simulink model "hoppingControl"  (R2018b)
settings: Solver=FixedStepAuto  StartTime=0.0  StopTime=inf  RelTol=1e-3  EnableMultiTasking=on
libraries: dspstat3 x19, cm_custom x9, raspberrypilib x8, simulink_extras x3, peGeneralControl x3, can_bus_multi x2, simulink x1, embdlinuxlib x1
(part 1 of 3)
settings Model: SimulationMode=external  Creator=Ivan Fan  LastModifiedBy=User
settings SolverCC: PositivePriorityOrder=on
settings OptimizationCC: EnhancedBackFolding=on  PassReuseOutputArgsThreshold=0  MaxStackSize=64  OptimizeBlockOrder=speed  DifferentSizesBufferReuse=on
settings DebuggingCC: ParameterTunabilityLossMsg=error  UnderSpecifiedDimensionMsg=error
settings HardwareCC: ProdBitPerPointer=32  ProdBitPerSizeT=32  ProdBitPerPtrDiffT=32  ProdLargestAtomicInteger=Long  ProdLargestAtomicFloat=Double  ProdWordSize=32  ProdHWDeviceType=ARM Compatible->ARM Cortex  UseEmbeddedCoderFeatures=off
settings SFSimCC: MATLABDynamicMemAlloc=off
settings RTWCC: SystemTargetFile=ert.tlc  HardwareBoard=Raspberry Pi  TLCOptions="-aInlineSetEventsForThisBaseRateFcn=TLC_FALSE -aSuppressMultiTaskScheduler=TLC_FALSE  -aRateBasedStepFcn=0"  TemplateMakefile=ert_default_tmf  GenerateReport=on  Toolchain=GNU GCC Raspberry Pi  BuildConfiguration=Faster Runs  LaunchReport=on  TargetLang=C++
settings CodeAppCC: ForceParamTrailComments=on  OperatorAnnotations=on
settings ERTTargetCC: TargetLangStandard=C++03 (ISO)  ERTCustomFileBanners=off  SupportContinuousTime=on  SupportNonInlinedSFcns=on  RemoveResetFunc=off  SupportVariableSizeSignals=on  ModelStepFunctionPrototypeControlCompliant=off  ExtMode=on  ExtModeMexArgs='192.168.137.181' 0 17725  ERTSrcFileBannerTemplate=codertarget_code_template.cgt  ERTHdrFileBannerTemplate=codertarget_code_template.cgt  ERTDataSrcFileTemplate=codertarget_code_template.cgt  ERTDataHdrFileTemplate=codertarget_code_template.cgt

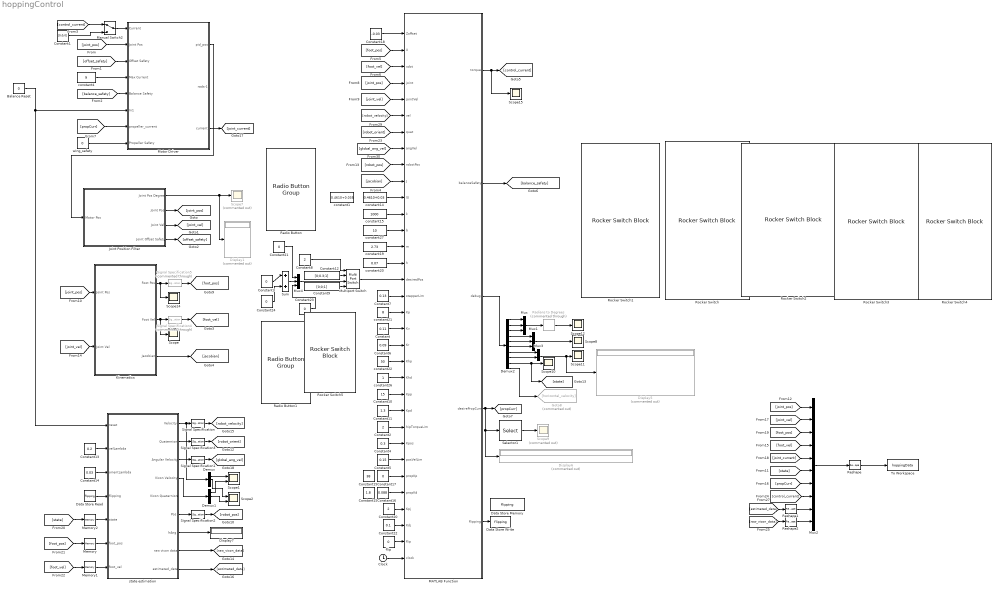
== system hoppingControl ==
  Balance Reset : Constant  Value=0
  Clock : Clock
  Constant : Constant  Value=0.11
  Constant1 : Constant  Value=[0;0;0]
  Constant10 : Constant  Value=15
  Constant11 : Constant  Value=1.3
  Constant12 : Constant  Value=[0;0.3;1]
  Constant13 : Constant  Value=0.2
  Constant14 : Constant  Value=0.03  VectorParams1D=off
  Constant15 : Constant  Value=1.8
  Constant16 : Constant  Value=0.088
  Constant{3,17,21,23..24} (5 alike) : Constant  Value=0
  Constant18 : Constant  Value=-0.03
  Constant19 : Constant  Value=38
  Constant2 : Constant  Value=2
  Constant20 : Constant  Value=2
  Constant22 : Constant  Value=0.1
  Constant4 : Constant  Value=0.3
  Constant5 : Constant  Value=0.15
  Constant6 : Constant  Value=0.09
  Constant7 : Constant  Value=0.13
  Constant8 : Constant  Value=2
  Constant9 : Constant  Value=[0;0;1]
  Data Store Memory : DataStoreMemory  DataStoreName=flipping  ReadBeforeWriteMsg=warning  WriteAfterWriteMsg=warning  WriteAfterReadMsg=warning  ShowAdditionalParam=off
  Data Store Read : DataStoreRead  DataStoreName=flipping
  Data Store Write : DataStoreWrite  DataStoreName=flipping
  Demux : Demux  Outputs=3
  Demux1 : Demux  Outputs=3
  Demux2 : Demux  Outputs=10
  Display1 : Display  Commented=on
      settings: Decimation=100
  Display5 : Display  Commented=on
  Display6 : Display  Commented=on
  Display7 : Display
  Goto8 : Goto  Commented=on  GotoTag=horizontal_velocity
  Joint Position Filter : Subsystem
  Kinematics : Subsystem
  MATLAB Function : MATLAB Function  TreatAsAtomicUnit=on
  Manual Switch2 : ManualSwitch
  Memory : Memory  InitialCondition=[0;0;0]
  Memory1 : Memory  InitialCondition=[0;0;0]
  Memory2 : Memory
  Motor Driver : Subsystem
  Multiport Switch : MultiPortSwitch
  Mux : Mux  Inputs=3
  Mux1 : Mux  Inputs=3
  Mux2 : Mux  Inputs=10
  Mux3 : Mux  Inputs=2
  Mux4 : Mux  Inputs=3
  Radians to Degrees : simulink_extras/Transformations/Radians to Degrees  Commented=through
  Radio Button : RadioButtonGroup  WebBlockId=1587  SelectedLabel=0  ButtonGroupName=x fine tune
      settings: Values={{'0.3', '0.2', '0.1', '0', '-0.1', '-0.2', '-0.3'}, [0.3 0.2 0.1 0 -0.1 -0.2 -0.3]}
  Radio Button1 : RadioButtonGroup  WebBlockId=1588  SelectedLabel=0  ButtonGroupName=y fine tune
      settings: Values={{'0.3', '0.2', '0.1', '0', '-0.1', '-0.2', '-0.3'}, [0.3 0.2 0.1 0 -0.1 -0.2 -0.3]}
  Reshape : Reshape
  Reshape1 : Reshape  OutputDimensionality=Column vector (2-D)
  Reshape2 : Reshape  OutputDimensionality=Column vector (2-D)
  Rocker Switch : RockerSwitchBlock  WebBlockId=606
      settings: Values={{'Off', 'On'}, [0 1]}
  Rocker Switch1 : RockerSwitchBlock  WebBlockId=618
      settings: Values={{'Off', 'On'}, [0 1]}
  Rocker Switch2 : RockerSwitchBlock  WebBlockId=667
      settings: Values={{'Off', 'On'}, [0 1]}
  Rocker Switch3 : RockerSwitchBlock  WebBlockId=1032
      settings: Values={{'Off', 'On'}, [0 1]}
  Rocker Switch4 : RockerSwitchBlock  WebBlockId=1024
      settings: Values={{'Off', 'On'}, [0 1]}
  Rocker Switch5 : RockerSwitchBlock  WebBlockId=1531
      settings: Values={{'Off', 'On'}, [-8 0]}
  Scope{,8,10..12,14..15} (7 alike) : Scope
  Scope1 : Scope  NumInputPorts=2
  Scope2 : Scope  NumInputPorts=2
  Scope7 : Scope  Commented=on
  Scope9 : Scope  Commented=on
  Selector1 : Selector  InputPortWidth=4  IndexOptions=Index vector (dialog)  Indices=[2 3 4]  OutputSizes=1
  Signal Specification : SignalSpecification  Dimensions=3
  Signal Specification1 : SignalSpecification  Dimensions=3
  Signal Specification2 : SignalSpecification  Dimensions=3
  Signal Specification3 : SignalSpecification  Dimensions=4
  Signal Specification4 : SignalSpecification  Commented=through  Dimensions=[3 1]
  Signal Specification5 : SignalSpecification  Commented=through  Dimensions=[3 1]
  Sum : Sum  Inputs=|++
  To Workspace : ToWorkspace  VariableName=hoppingData  SampleTime=-1
      settings: Save2DSignal=2-D array (concatenate along first dimension)
  constant1 : Constant  Value=0.4610+0.035
  constant14 : Constant  Value=0.4610+0.03
  constant15 : Constant  Value=1000
  constant19 : Constant  Value=2.73
  constant20 : Constant  Value=0.07
  constant21 : Constant  Value=8
  constant22 : Constant  Value=50
  constant26 : Constant
  constant27 : Constant  Value=10
  constant4 : Constant  Value=9
  flip : Constant  Value=0
  state estimation : Subsystem
  wing_safety : Constant  Value=0
  wires:
  Constant1/1 -> Manual Switch2/2
  Manual Switch2/1 -> Motor Driver/1(Current)
  Joint Position Filter/1(Joint Pos Degree) -> Scope7/1, Display1/1
  Joint Position Filter/2(Joint Pos) -> [joint_pos]
  Joint Position Filter/3(Joint Vel) -> [joint_vel]
  [joint_pos] -> Motor Driver/2(Joint Pos)
  [offset_safety] -> Motor Driver/3(Offset Safety)
  constant4/1 -> Motor Driver/4(Max Current)
  [balance_safety] -> Motor Driver/5(Balance Safety)
  [control_current] -> Manual Switch2/1
  Kinematics/2(Foot Vel) -> Signal Specification4/1, Scope/1
  [joint_pos] -> Kinematics/1(Joint Pos)
  [joint_vel] -> Kinematics/2(Joint Vel)
  [jacobian] -> MATLAB Function/10(J)
  [foot_pos] -> MATLAB Function/2(X)
  Constant18/1 -> MATLAB Function/1(Zoffset)
  [foot_vel] -> MATLAB Function/3(xdot)
  constant14/1 -> MATLAB Function/11(l0)
  constant27/1 -> MATLAB Function/13(b)
  constant15/1 -> MATLAB Function/12(k)
  constant19/1 -> MATLAB Function/14(m)
  constant20/1 -> MATLAB Function/15(h)
  Constant7/1 -> MATLAB Function/17(stepperLim)
  constant21/1 -> MATLAB Function/18(Kp)
  constant22/1 -> MATLAB Function/21(Khp)
  constant26/1 -> MATLAB Function/22(Khd)
  Constant6/1 -> MATLAB Function/20(Kr)
  Constant/1 -> MATLAB Function/19(Kv)
  MATLAB Function/1(torque) -> Scope15/1, [control_current]
  MATLAB Function/2(balanceSafety) -> [balance_safety]
  Kinematics/3(Jacobian) -> [jacobian]
  Constant10/1 -> MATLAB Function/23(Kpp)
  Constant11/1 -> MATLAB Function/24(Kpd)
  Constant2/1 -> MATLAB Function/25(hipTorqueLim)
  Balance Reset/1 -> Motor Driver/6(In1), state estimation/1(reset)
  MATLAB Function/3(debug) -> Demux2/1
  state estimation/4(Vicon Velocity) -> Demux1/1
  Demux/1 -> Scope1/1
  Demux1/1 -> Scope1/2
  Demux/2 -> Scope2/1
  Demux1/2 -> Scope2/2
  Constant4/1 -> MATLAB Function/26(Kpos)
  Constant5/1 -> MATLAB Function/27(posVelLim)
  Constant8/1 -> Multiport Switch/1
  Constant9/1 -> Multiport Switch/4
  Constant12/1 -> Multiport Switch/2
  Constant14/1 -> state estimation/3(orientLambda)
  Constant13/1 -> state estimation/2(velLambda)
  [propCurr] -> Motor Driver/7(propeller_current)
  Constant17/1 -> MATLAB Function/28(propKp)
  Demux2/5 -> Mux1/2
  Demux2/4 -> Mux1/1
  Demux2/3 -> Mux/3
  Demux2/2 -> Mux/2
  Demux2/1 -> Mux/1
  Mux/1 -> Radians to Degrees/1
  Constant16/1 -> MATLAB Function/29(propKd)
  Demux2/6 -> Mux1/3
  Multiport Switch/1 -> MATLAB Function/16(desiredPos)
  Demux2/9 -> [state], Scope10/1
  Demux2/7 -> Mux3/1
  Demux2/8 -> Mux3/2
  Demux2/10 -> Goto8/1
  MATLAB Function/4(desirePropCurr) -> Display6/1, Selector1/1, [propCurr]
  [joint_pos] -> MATLAB Function/4(joint)
  [joint_vel] -> MATLAB Function/5(jointVel)
  Clock/1 -> MATLAB Function/33(clock)
  Constant20/1 -> MATLAB Function/30(Kpj)
  Constant22/1 -> MATLAB Function/31(Kdj)
  Mux1/1 -> Scope8/1
  wing_safety/1 -> Motor Driver/8(Propeller Safety)
  flip/1 -> MATLAB Function/32(flip)
  MATLAB Function/5(flipping) -> Data Store Write/1
  Data Store Read/1 -> state estimation/4(flipping)
  Radians to Degrees/1 -> Scope12/1
  Selector1/1 -> Scope9/1
  Mux3/1 -> Display5/1, Scope11/1
  [robot_pos] -> MATLAB Function/9(robotPos)
  [joint_pos] -> Mux2/1
  [joint_vel] -> Mux2/2
  Mux2/1 -> Reshape/1
  [state] -> Mux2/6
  Joint Position Filter/4(Joint Offset Safety) -> [offset_safety]
  Motor Driver/1(pid_pos) -> Joint Position Filter/1(Motor Pos)
  [foot_pos] -> Mux2/3
  [state] -> Memory2/1
  [foot_pos] -> Memory/1
  [foot_vel] -> Memory1/1
  Kinematics/1(Foot Pos) -> Signal Specification5/1, Scope14/1
  Memory/1 -> state estimation/6(foot_pos)
  Memory1/1 -> state estimation/7(foot_vel)
  Memory2/1 -> state estimation/5(state)
  state estimation/6(Pos) -> Signal Specification2/1
  state estimation/3(Angular Velocity) -> Signal Specification1/1
  state estimation/1(Velocity) -> Demux/1, Signal Specification/1
  state estimation/2(Quaternion) -> Signal Specification3/1
  Signal Specification/1 -> [robot_velocity]
  Signal Specification1/1 -> [global_ang_vel]
  Signal Specification2/1 -> [robot_pos]
  Signal Specification3/1 -> [robot_orient]
  [robot_orient] -> MATLAB Function/7(quat)
  Signal Specification4/1 -> [foot_vel]
  Signal Specification5/1 -> [foot_pos]
  state estimation/7(hAng) -> Display7/1
  state estimation/8(raw vicon data) -> [raw_vicon_data]
  [control_current] -> Mux2/8
  Reshape/1 -> To Workspace/1
  [raw_vicon_data] -> Reshape2/1
  state estimation/9(estimated_data) -> [estimated_data]
  [estimated_data] -> Reshape1/1
  Motor Driver/3(current) -> [joint_current]
  Constant23/1 -> Mux4/3
  Constant21/1 -> Mux4/1
  Constant3/1 -> Sum/1
  Mux4/1 -> Multiport Switch/3
  [robot_velocity] -> MATLAB Function/6(vel)
  [global_ang_vel] -> MATLAB Function/8(angVel)
  [foot_vel] -> Mux2/4
  [propCurr] -> Mux2/7
  [joint_current] -> Mux2/5
  Reshape1/1 -> Mux2/9
  Reshape2/1 -> Mux2/10
  Constant24/1 -> Sum/2
  Sum/1 -> Mux4/2

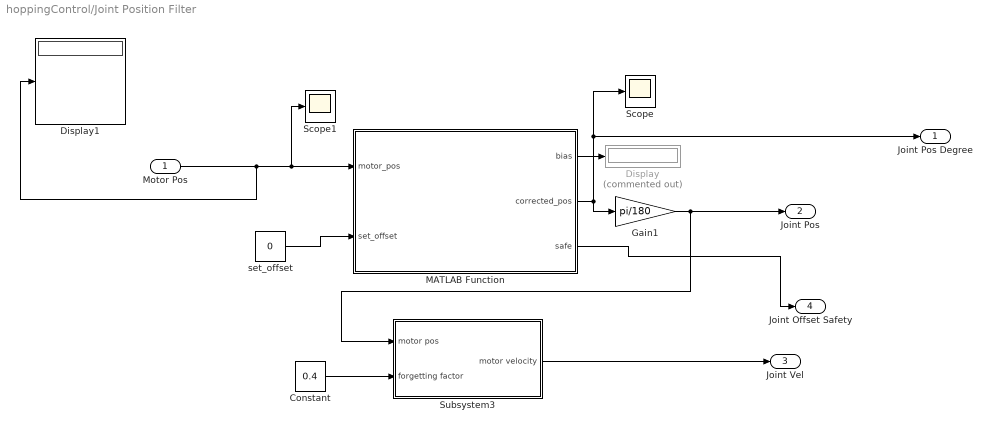
== system hoppingControl/Joint Position Filter ==
  Motor Pos : Inport
  Constant : Constant  Value=0.4
  Display : Display  Commented=on
      settings: Decimation=100
  Display1 : Display
  Gain1 : Gain  Gain=pi/180
  MATLAB Function : MATLAB Function  TreatAsAtomicUnit=on
  Scope : Scope
  Scope1 : Scope
  Subsystem3 : Subsystem
  set_offset : Constant  Value=0
  Joint Pos Degree : Outport
  Joint Pos : Outport  Port=2
  Joint Vel : Outport  Port=3
  Joint Offset Safety : Outport  Port=4
  wires:
  Subsystem3/1("motor velocity ") -> Joint Vel/1
  MATLAB Function/2(corrected_pos) -> Scope/1, Joint Pos Degree/1, Gain1/1
  MATLAB Function/1(bias) -> Display/1
  set_offset/1 -> MATLAB Function/2(set_offset)
  Constant/1 -> Subsystem3/2(forgetting factor)
  Motor Pos/1 -> Display1/1, Scope1/1, MATLAB Function/1(motor_pos)
  MATLAB Function/3(safe) -> Joint Offset Safety/1
  Gain1/1 -> Subsystem3/1(motor pos), Joint Pos/1

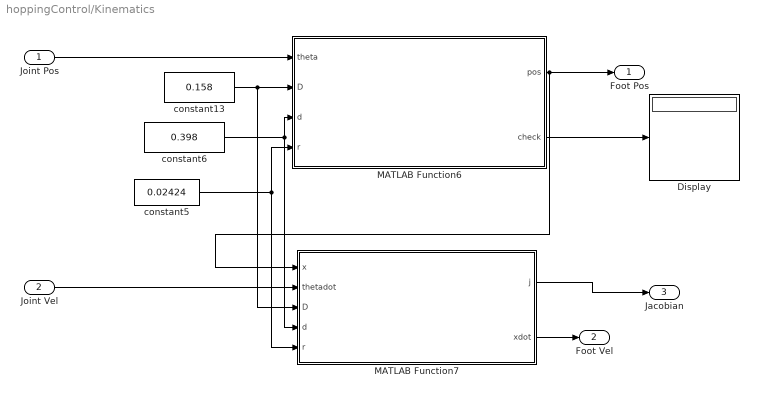
== system hoppingControl/Kinematics ==
  Joint Pos : Inport
  Joint Vel : Inport  Port=2
  Display : Display
      settings: Decimation=100
  MATLAB Function6 : MATLAB Function  TreatAsAtomicUnit=on
  MATLAB Function7 : MATLAB Function  TreatAsAtomicUnit=on
  constant13 : Constant  Value=0.158
  constant5 : Constant  Value=0.02424
  constant6 : Constant  Value=0.398
  Foot Pos : Outport
  Foot Vel : Outport  Port=2
  Jacobian : Outport  Port=3
  wires:
  constant6/1 -> MATLAB Function7/4(d), MATLAB Function6/3(d)
  constant5/1 -> MATLAB Function7/5(r), MATLAB Function6/4(r)
  constant13/1 -> MATLAB Function6/2(D), MATLAB Function7/3(D)
  Joint Pos/1 -> MATLAB Function6/1(theta)
  MATLAB Function7/1(j) -> Jacobian/1
  MATLAB Function6/2(check) -> Display/1
  Joint Vel/1 -> MATLAB Function7/2(thetadot)
  MATLAB Function6/1(pos) -> MATLAB Function7/1(x), Foot Pos/1
  MATLAB Function7/2(xdot) -> Foot Vel/1

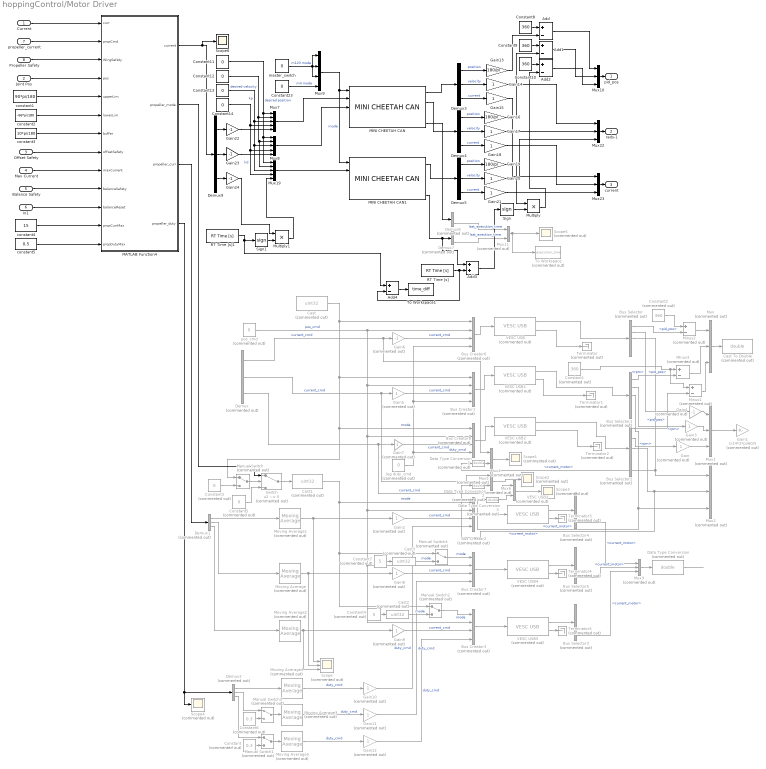
== system hoppingControl/Motor Driver ==
  Current : Inport
  Joint Pos : Inport  Port=2
  Offset Safety : Inport  Port=3
  Max Current : Inport  Port=4
  Balance Safety : Inport  Port=5
  In1 : Inport  Port=6
  propeller_current : Inport  Port=7
  Propeller Safety : Inport  Port=8
  Add{,1..2,4} (4 alike) : Sum  Inputs=+-
  Add3 : Sum
  Bus Creator{1..3,6..8} (6 alike) : BusCreator  Commented=on  Inputs=4
  Bus Selector : BusSelector  Commented=on  OutputSignals=pid_pos,rpm,current_motor,v_in,fault_code
  Bus Selector1 : BusSelector  Commented=on  OutputSignals=pid_pos,rpm,current_motor,v_in,fault_code
  Bus Selector2 : BusSelector  Commented=on  OutputSignals=pid_pos,rpm,current_motor,v_in,fault_code
  Bus Selector3 : BusSelector  Commented=on  OutputSignals=pid_pos,rpm,current_motor
  Bus Selector4 : BusSelector  Commented=on  OutputSignals=pid_pos,rpm,current_motor
  Bus Selector5 : BusSelector  Commented=on  OutputSignals=pid_pos,rpm,current_motor
  Cast{,1..3} (4 alike) : DataTypeConversion  Commented=on  OutDataTypeStr=uint32  RndMeth=Round
  Cast To Double : DataTypeConversion  Commented=on  OutDataTypeStr=double
  Constant : Constant  Commented=on  Value=0.3
  Constant1 : Constant  Commented=on  Value=360  OutDataTypeStr=Inherit: Inherit via back propagation
  Constant10 : Constant  Value=360
  Constant{11..14,23} (5 alike) : Constant  Value=0
  Constant2 : Constant  Commented=on  Value=360  OutDataTypeStr=Inherit: Inherit via back propagation
  Constant3 : Constant  Commented=on  Value=0
  Constant4 : Constant  Commented=on  Value=5
  Constant5 : Constant  Commented=on  Value=0
  Constant6 : Constant  Commented=on  Value=0.3
  Constant7 : Constant  Commented=on  Value=5
  Constant8 : Constant  Value=360
  Constant9 : Constant  Value=360
  Data Type Conversion{,1..3} (4 alike) : DataTypeConversion  Commented=on  OutDataTypeStr=double
  Demux{,1..2,7..8} (5 alike) : Demux  Commented=on  Outputs=3
  Demux{3..5,9} (4 alike) : Demux  Outputs=3
  Gain{,3,5,7} (4 alike) : Gain  Commented=on  OutDataTypeStr=Inherit: Same as input
  Gain1 : Gain  Commented=on  Gain=1/14*2*pi/60/5  OutDataTypeStr=Inherit: Same as input
  Gain{2,8..12} (6 alike) : Gain  Commented=on
  Gain13 : Gain  Gain=180/pi
  Gain{14..15,17..18,20..21} (6 alike) : Gain
  Gain16 : Gain  Gain=180/pi
  Gain19 : Gain  Gain=180/pi
  Gain22 : Gain  Gain=-1
  Gain23 : Gain  Gain=-1
  Gain24 : Gain  Gain=-1
  Gain4 : Gain  Commented=on  Gain=-1  OutDataTypeStr=Inherit: Same as input
  Gain6 : Gain  Commented=on  Gain=-1  OutDataTypeStr=Inherit: Same as input
  MATLAB Function4 : MATLAB Function  TreatAsAtomicUnit=on
  MINI CHEETAH CAN : can_bus_multi/MINI CHEETAH CAN  PAR_PORT_NUM=can0  PAR_SAFE=on  PAR_DEV_NUM=3  PAR_SMPLT=0.002
      link override S-Function Builder: Parameters=uint8(PAR_DEV_NUM),uint8(PAR_PORT_NUM),uint8(PAR_SAFE)  FunctionName=CAN_BUS_MULTISTATE_SF  SFunctionModules=CAN_BUS_MULTISTATE_SF_wrapper
      settings: SourceProductName=CAN Bus Multi
  MINI CHEETAH CAN1 : can_bus_multi/MINI CHEETAH CAN  PAR_PORT_NUM=can1  PAR_SAFE=on  PAR_DEV_NUM=1  PAR_SMPLT=0.002
      link override S-Function Builder: Parameters=uint8(PAR_DEV_NUM),uint8(PAR_PORT_NUM),uint8(PAR_SAFE)  FunctionName=CAN_BUS_MULTISTATE_SF  SFunctionModules=CAN_BUS_MULTISTATE_SF_wrapper
      settings: SourceProductName=CAN Bus Multi
  Manual Switch{,1..4} (5 alike) : ManualSwitch  Commented=on
  Minus1 : Sum  Commented=on  Inputs=+-
  Minus2 : Sum  Commented=on  Inputs=+-
  Minus3 : Sum  Commented=on  Inputs=+-
  Moving Average{,1..5} (6 alike) : dspstat3/Moving Average  Commented=on  Method=Sliding window  ForgettingFactorPort=off  SpecifyWindowLength=on  WindowLength=4  ForgettingFactor=0.9  SimulateUsing=Code generation
  Multiply : Product
  Multiply1 : Product
  Mux{,1..3} (4 alike) : Mux  Commented=on  Inputs=3
  Mux10 : Mux  Inputs=3
  Mux{4..6,11} (4 alike) : Mux  Commented=on  Inputs=2
  Mux19 : Mux  Inputs=5
  Mux22 : Mux  Inputs=3
  Mux23 : Mux  Inputs=3
  Mux7 : Mux  Inputs=5
  Mux8 : Mux  Inputs=5
  Mux9 : Mux
  RT Time [s] : cm_custom/RT Time [s]
      settings: SourceProductName=cm custom
  RT Time [s]1 : cm_custom/RT Time [s]
      settings: SourceProductName=cm custom
  Scope : Scope  Commented=on  NumInputPorts=3
  Scope{1..5} (5 alike) : Scope  Commented=on
  Scope6 : Scope
  Sign : Signum
  Sign1 : Signum
  Switch : Switch  Commented=on  Criteria=u2 ~= 0
  Terminator{,1..5} (6 alike) : Terminator  Commented=on
  To Workspace : ToWorkspace  Commented=on  VariableName=execution_time  SampleTime=-1
  To Workspace1 : ToWorkspace  VariableName=time_diff  SampleTime=-1
      settings: Save2DSignal=2-D array (concatenate along first dimension)
  VESC USB : cm_custom/VESC USB  Commented=on  PAR_VESC_DEV='/dev/leg_a'  POS_KP=0.05  POS_KI=0  POS_KD=0.0008  POS_KD_FIL=0.8  POS_DIV=5  CURR_MAX=25  CURR_MIN=-25  CURR_IN_MAX=20  CURR_IN_MIN=-20  CURR_ABS_MAX=40  PAR_SMPLT=0.0015
      link override S-Function Builder5: Parameters=uint8(PAR_VESC_DEV)
      settings: SourceProductName=cm custom
  VESC USB1 : cm_custom/VESC USB  Commented=on  PAR_VESC_DEV='/dev/leg_b'  POS_KP=0.05  POS_KI=0  POS_KD=0.0008  POS_KD_FIL=0.8  POS_DIV=5  CURR_MAX=25  CURR_MIN=-25  CURR_IN_MAX=20  CURR_IN_MIN=-20  CURR_ABS_MAX=40  PAR_SMPLT=0.0015
      settings: SourceProductName=cm custom
  VESC USB2 : cm_custom/VESC USB  Commented=on  PAR_VESC_DEV='/dev/leg_c'  POS_KP=0.05  POS_KI=0  POS_KD=0.0008  POS_KD_FIL=0.8  POS_DIV=5  CURR_MAX=25  CURR_MIN=-25  CURR_IN_MAX=20  CURR_IN_MIN=-20  CURR_ABS_MAX=40  PAR_SMPLT=0.0015
      link override S-Function Builder5: Parameters=uint8(PAR_VESC_DEV)
      settings: SourceProductName=cm custom
  VESC USB3 : cm_custom/VESC USB  Commented=on  PAR_VESC_DEV='/dev/wing_a'  POS_KP=0.03  POS_KI=0  POS_KD=0.0004  POS_KD_FIL=0.2  POS_DIV=1  CURR_MAX=42  CURR_MIN=-42  CURR_IN_MAX=42  CURR_IN_MIN=-42  CURR_ABS_MAX=130  PAR_SMPLT=0.0015
      settings: SourceProductName=cm custom
  VESC USB4 : cm_custom/VESC USB  Commented=on  PAR_VESC_DEV='/dev/wing_b'  POS_KP=0.03  POS_KI=0  POS_KD=0.0004  POS_KD_FIL=0.2  POS_DIV=1  CURR_MAX=42  CURR_MIN=-42  CURR_IN_MAX=99  CURR_IN_MIN=-60  CURR_ABS_MAX=130  PAR_SMPLT=0.0015
      link override S-Function Builder5: Parameters=uint8(PAR_VESC_DEV)
      settings: SourceProductName=cm custom
  VESC USB5 : cm_custom/VESC USB  Commented=on  PAR_VESC_DEV='/dev/wing_c'  POS_KP=0.03  POS_KI=0  POS_KD=0.0004  POS_KD_FIL=0.2  POS_DIV=1  CURR_MAX=42  CURR_MIN=-42  CURR_IN_MAX=99  CURR_IN_MIN=-60  CURR_ABS_MAX=130  PAR_SMPLT=0.0015
      settings: SourceProductName=cm custom
  constant1 : Constant  Value=90*pi/180
  constant2 : Constant  Value=-66*pi/180
  constant3 : Constant  Value=10*pi/180
  constant4 : Constant  Value=15
  constant5 : Constant  Value=0.5
  leg duty_cmd : Constant  Commented=on  Value=0
  master_switch : Constant  Value=0  OutDataTypeStr=double
  pos_cmd : Constant  Commented=on  Value=0
  pid_pos : Outport
  rads-1 : Outport  Port=2
  current : Outport  Port=3
  wires:
  Bus Creator6/1 -> VESC USB/1
  Bus Creator1/1 -> VESC USB1/1
  Bus Creator8/1 -> VESC USB2/1
  Demux/1 -> Mux4/1, Gain6/1  "current_cmd"
  VESC USB/1 -> Bus Selector/1
  VESC USB1/1 -> Bus Selector1/1
  VESC USB2/1 -> Bus Selector2/1
  VESC USB/2 -> Terminator/1
  VESC USB1/2 -> Terminator1/1
  VESC USB2/2 -> Terminator2/1
  Bus Selector2/1 -> Minus1/2  "<pid_pos>"
  Bus Selector/2 -> Gain4/1  "<rpm>"
  Bus Selector2/2 -> Gain/1  "<rpm>"
  Bus Selector1/2 -> Gain3/1  "<rpm>"
  Bus Selector/3 -> Mux2/1, Data Type Conversion1/1  "<current_motor>"
  Mux/1 -> Cast To Double/1
  Mux1/1 -> Gain1/1
  Constant1/1 -> Minus3/1, Minus1/1
  Gain4/1 -> Mux1/1
  Gain6/1 -> Bus Creator6/3  "current_cmd"
  Bus Selector2/3 -> Data Type Conversion2/1, Mux2/2  "<current_motor>"
  Bus Selector1/3 -> Data Type Conversion3/1, Mux2/3  "<current_motor>"
  Bus Selector/1 -> Minus2/2  "<pid_pos>"
  Minus2/1 -> Mux/1
  Constant2/1 -> Minus2/1
  Gain/1 -> Mux1/3
  Gain3/1 -> Mux1/2
  Demux/2 -> Mux5/1, Gain5/1  "current_cmd"
  Demux/3 -> Mux6/1, Gain7/1  "current_cmd"
  Bus Selector1/1 -> Minus3/2  "<pid_pos>"
  Minus3/1 -> Mux/2
  Minus1/1 -> Mux/3
  Current/1 -> MATLAB Function4/1(curr)
  Joint Pos/1 -> MATLAB Function4/4(pos)
  constant1/1 -> MATLAB Function4/5(upperLim)
  constant2/1 -> MATLAB Function4/6(lowerLim)
  constant3/1 -> MATLAB Function4/7(buffer)
  Offset Safety/1 -> MATLAB Function4/8(offsetSafety)
  Max Current/1 -> MATLAB Function4/9(maxCurrent)
  Balance Safety/1 -> MATLAB Function4/10(balanceSafety)
  In1/1 -> MATLAB Function4/11(balanceReset)
  Bus Creator2/1 -> VESC USB3/1
  Bus Creator7/1 -> VESC USB4/1
  VESC USB4/2 -> Terminator4/1
  VESC USB3/2 -> Terminator3/1
  Demux1/1 -> Moving Average1/1
  Demux1/2 -> Moving Average/1
  propeller_current/1 -> MATLAB Function4/2(propCmd)
  MATLAB Function4/3(propeller_curr) -> Demux1/1
  Moving Average1/1 -> Scope/1, Gain2/1
  Moving Average/1 -> Scope/2, Gain8/1
  VESC USB3/1 -> Bus Selector4/1
  VESC USB4/1 -> Bus Selector5/1
  Bus Selector5/3 -> Mux3/2  "<current_motor>"
  Bus Selector4/3 -> Mux3/1  "<current_motor>"
  Mux3/1 -> Data Type Conversion/1
  Data Type Conversion/1 -> ?
  Bus Creator3/1 -> VESC USB5/1
  Moving Average2/1 -> Scope/3, Gain9/1
  Demux1/3 -> Moving Average2/1
  VESC USB5/1 -> Bus Selector3/1
  VESC USB5/2 -> Terminator5/1
  Bus Selector3/3 -> Mux3/3  "<current_motor>"
  Gain5/1 -> Bus Creator1/3  "current_cmd"
  Gain7/1 -> Bus Creator8/3  "current_cmd"
  Cast/1 -> Bus Creator1/1, Manual Switch/1, Bus Creator8/1, Bus Creator6/1  "mode"
  leg duty_cmd/1 -> Bus Creator6/4, Bus Creator1/4, Bus Creator8/4  "duty_cmd"
  pos_cmd/1 -> Bus Creator3/2, Bus Creator7/2, Bus Creator2/2, Bus Creator8/2, Bus Creator1/2, Bus Creator6/2  "pos_cmd"
  Cast1/1 -> Manual Switch2/1, Manual Switch4/1, Bus Creator2/1  "mode"
  MATLAB Function4/2(propeller_mode) -> Switch/1
  Constant5/1 -> Switch/3
  Switch/1 -> Cast1/1
  Gain9/1 -> Bus Creator3/3  "current_cmd"
  Gain8/1 -> Bus Creator7/3  "current_cmd"
  Gain2/1 -> Bus Creator2/3  "current_cmd"
  constant4/1 -> MATLAB Function4/12(propCurrMax)
  constant5/1 -> MATLAB Function4/13(propDutyMax)
  Demux2/3 -> Manual Switch1/1
  Moving Average4/1 -> Gain10/1  "duty_cmd"
  Demux2/2 -> Manual Switch3/1
  Demux2/1 -> Moving Average4/1
  MATLAB Function4/4(propeller_duty) -> Scope4/1, Demux2/1
  Moving Average3/1 -> Gain11/1  "duty_cmd"
  Moving Average5/1 -> Gain12/1  "duty_cmd"
  Gain10/1 -> Bus Creator2/4  "duty_cmd"
  Gain11/1 -> Bus Creator7/4  "duty_cmd"
  Gain12/1 -> Bus Creator3/4  "duty_cmd"
  Manual Switch/1 -> Switch/2
  Constant3/1 -> Manual Switch/2
  Mux4/1 -> Scope1/1
  Mux5/1 -> Scope2/1
  Mux6/1 -> Scope3/1
  Data Type Conversion1/1 -> Mux4/2
  Data Type Conversion2/1 -> Mux5/2
  Data Type Conversion3/1 -> Mux6/2
  Manual Switch2/1 -> Bus Creator3/1  "mode"
  Manual Switch1/1 -> Moving Average5/1
  Constant/1 -> Manual Switch1/2
  Constant4/1 -> Cast2/1
  Cast2/1 -> Manual Switch2/2  "mode"
  Propeller Safety/1 -> MATLAB Function4/3(WingSafety)
  Constant6/1 -> Manual Switch3/2
  Manual Switch3/1 -> Moving Average3/1
  Cast3/1 -> Manual Switch4/2  "mode"
  Constant7/1 -> Cast3/1
  Manual Switch4/1 -> Bus Creator7/1  "mode"
  Mux8/1 -> MINI CHEETAH CAN/3
  MATLAB Function4/1(current) -> Scope6/1, Demux9/1
  Mux7/1 -> MINI CHEETAH CAN/2
  Constant14/1 -> Mux7/4, Mux8/4, Mux19/4  "kd"
  Constant13/1 -> Mux8/3, Mux19/3, Mux7/3  "kp"
  Demux9/2 -> Gain23/1
  Demux9/1 -> Gain22/1
  master_switch/1 -> Mux9/3, Mux9/1, Mux9/2  "m123 mode"
  Constant11/1 -> Mux19/1, Mux8/1, Mux7/1  "desired position"
  Mux19/1 -> MINI CHEETAH CAN1/2
  Gain23/1 -> Mux8/5
  Constant23/1 -> Mux9/4  "m4 mode"
  Constant12/1 -> Mux7/2, Mux19/2, Mux8/2  "desired velocity"
  Gain22/1 -> Mux7/5
  Demux9/3 -> Gain24/1
  Mux9/1 -> MINI CHEETAH CAN/1, MINI CHEETAH CAN1/1  "mode"
  Demux5/1 -> Gain19/1  "position"
  Constant8/1 -> Add/1
  Gain17/1 -> Mux22/2
  Gain16/1 -> Add1/2
  Mux10/1 -> pid_pos/1
  Demux3/3 -> Gain15/1  "current"
  Constant10/1 -> Add2/1
  Gain21/1 -> Mux23/3
  Constant9/1 -> Add1/1
  Add/1 -> Mux10/1
  Demux5/3 -> Gain21/1  "current"
  Demux5/2 -> Gain20/1  "velocity"
  Demux4/2 -> Gain17/1  "velocity"
  Demux4/3 -> Gain18/1  "current"
  Mux22/1 -> rads-1/1
  Demux3/1 -> Gain13/1  "position"
  Gain14/1 -> Mux22/1
  MINI CHEETAH CAN/2 -> Demux4/1
  MINI CHEETAH CAN/1 -> Demux3/1
  Gain18/1 -> Mux23/2
  Add1/1 -> Mux10/2
  Add2/1 -> Mux10/3
  MINI CHEETAH CAN1/1 -> Demux5/1
  Gain15/1 -> Mux23/1
  Demux4/1 -> Gain16/1  "position"
  Gain13/1 -> Add/2
  Demux3/2 -> Gain14/1  "velocity"
  MINI CHEETAH CAN/4 -> Demux8/1
  Demux7/3 -> Mux11/2  "last_exeution_time"
  Demux8/3 -> Mux11/1  "last_execution_time"
  Mux11/1 -> To Workspace/1, Scope5/1
  RT Time [s]/1 -> Add4/2, Add3/2
  MINI CHEETAH CAN1/4 -> Add3/1, Demux7/1
  Add3/1 -> Sign/1
  Sign/1 -> Multiply/2
  Gain20/1 -> Mux22/3
  Sign1/1 -> Multiply1/2
  Gain24/1 -> Multiply1/1
  RT Time [s]1/1 -> Add4/1, Sign1/1
  Multiply1/1 -> Mux19/5
  Multiply/1 -> Add2/2
  Gain19/1 -> Multiply/1
  Add4/1 -> To Workspace1/1
  Mux23/1 -> current/1

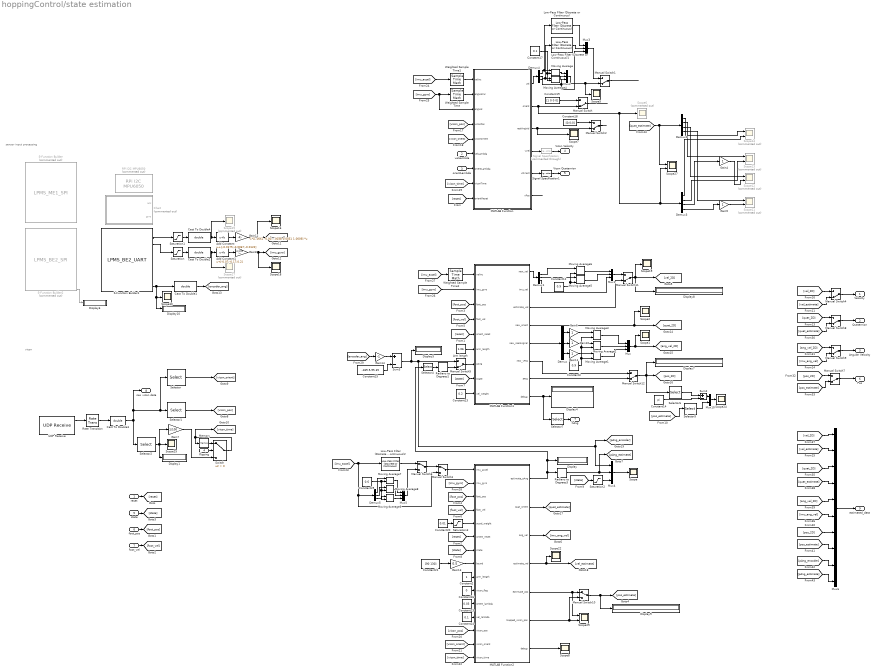
== system hoppingControl/state estimation ==
  note: vicon
  note: sensor input processing
  reset : Inport
  velLambda : Inport  Port=2
  orientLambda : Inport  Port=3
  flipping : Inport  Port=4
  state : Inport  Port=5
  foot_pos : Inport  Port=6
  foot_vel : Inport  Port=7
  Add Constant : Bias  Bias=-[-0.0175;-0.0067;-0.0122]
  Add Constant1 : Bias  Bias=[-0.07;-0.17;0.2]
  Arm length : Constant  Value=1.06
  Cast To Double{1..4} (4 alike) : DataTypeConversion  OutDataTypeStr=double
  Chart : Stateflow chart  Commented=on  TreatAsAtomicUnit=on  mask{PAR_SMPLT=0.002}
      mask prompts: PAR_SMPLT "Sampling Time [s]"
  Constant12 : Constant  Value=0.9
  Constant13 : Constant  Value=0.2
  Constant14 : Constant  Value=pi
  Constant15 : Constant  Value=-189.5-95.35
  Constant16 : Constant  Value=0
  Constant17 : Constant  Value=0.1
  Constant18 : Constant  Value=[0;0;0]
  Constant19 : Constant  Value=[1 0 0 0]  VectorParams1D=off
  Constant2 : Constant
  Constant20 : Constant  Value=0.01
  Constant21 : Constant  Value=[90 130]  VectorParams1D=off
  Constant23 : Constant  Value=0.03
  Constant24 : Constant  Value=0.1
  Constant25 : Constant  Value=0.6
  Constant3 : Constant  Value=0.9
  Demux{,1,4..5} (4 alike) : Demux  Outputs=3
  Demux2 : Demux
  Demux3 : Demux
  Display{,1,4..10} (9 alike) : Display
      Display1 settings: Decimation=100
      Display10 settings: Decimation=100
      Display6 settings: Decimation=100
  Gain{4..6,10..11} (5 alike) : Gain
  Gain12 : Gain  Gain=-1*[1.0061 -0.0076 0.0018; 0.0045 0.9996 0.0047; -0.0038 0.0031 1.0009]  Multiplication=Matrix(K*u)
  Gain13 : Gain  Gain=0.5
  Gain14 : Gain  Gain=-1
  Gain7 : Gain  Gain=1/100
  Gain8 : Gain  Gain=pi/180  Multiplication=Matrix(K*u)
  Low-Pass Filter (Discrete or Continuous) : peGeneralControl/Low-Pass Filter (Discrete or Continuous)  K=1  T=0.05  B=inf  A=-inf  Ts=-1
  Low-Pass Filter (Discrete or Continuous)1 : peGeneralControl/Low-Pass Filter (Discrete or Continuous)  K=1  T=0.05  B=inf  A=-inf  Ts=-1
  Low-Pass Filter (Discrete or Continuous)2 : peGeneralControl/Low-Pass Filter (Discrete or Continuous)  K=1  T=0.1  B=inf  A=-inf  Ts=-1
  MATLAB Function : MATLAB Function  TreatAsAtomicUnit=on
  MATLAB Function1 : MATLAB Function  TreatAsAtomicUnit=on
  MATLAB Function2 : MATLAB Function  TreatAsAtomicUnit=on
  Manual Switch{,1..2,4..5,7..9,11..12} (10 alike) : ManualSwitch  CurrentSetting=0
  Manual Switch10 : ManualSwitch
  Manual Switch3 : ManualSwitch
  Manual Switch6 : ManualSwitch
  Memory : Memory
  Moving Average{,1..9} (10 alike) : dspstat3/Moving Average  Method=Exponential weighting  ForgettingFactorPort=on  SpecifyWindowLength=on  WindowLength=4  ForgettingFactor=0.9  SimulateUsing=Code generation
  Mux{,1..5} (6 alike) : Mux  Inputs=3
  Mux10 : Mux  Inputs=2
  Mux6 : Mux  Inputs=10
  RPi I2C MPU6050 : cm_custom/RPi I2C MPU6050  Commented=on  PAR_SENS_ACC=([9.81 9.81 9.81] - [-9.81 -9.81 -9.81]) / 2 / 8192  PAR_SENS_GYRO=[1 1 1] * pi / 180 / 16.4  PAR_OFFSET_ACC=-[0 0 0]  PAR_OFFSET_GYRO=[0 0 0]  PAR_SMPLT=0.002
      settings: SourceProductName=cm custom
  Radians to Degrees1 : simulink_extras/Transformations/Radians to Degrees
  Radians to Degrees3 : simulink_extras/Transformations/Radians to Degrees
  Rate Transition : RateTransition  Deterministic=off  InitialCondition=[0 0 0 0 0 0 0]
  S-Function Builder : S-Function  Commented=on  InitFcn=try, set_param(gcb,'FunctionName','LPMS_ME1_SPI'), end  FunctionName=LPMS_ME1_SPI  SFunctionModules=LPMS_ME1_SPI_wrapper  SFunctionDeploymentMode=off  EnableBusSupport=off  mask(S-Function Builder){}
      mask help: Simulink:masks:SFunctionBuilder_MD
      mask init:
      | val = [[.9  0.75 0.75 1 1 .9 .9 1]',[1 1 0.75 0.75 .9 .9 1 .9]'];try , sys = get_param(gcb,'SfunBuilderFcnName');if isempty(sys), sys = get_param(gcb,'FunctionName'); end,catch, sys = get_param(gcb,'FunctionName'); end
      settings: CopyFcn=set_param(gcbh,'LinkStatus','none')  PreSaveFcn=try, set_param(gcb,'FunctionName','LPMS_ME1_SPI'), end  OpenFcn=sfunctionwizard(gcbh)
      mask Display: plot(val(:,1),val(:,2)),disp(sys), port_label('output',1,'config'), port_label('output',2,'acc'), port_label('output',3,'gyr'), port_label('output',4,'mag'), port_label('output',5,'euler'), port_label('output',6,'quat'), port_label('output',7,'lin_acc'), port_label('output',8,'temp'), port_label('output',9,'time')
  S-Function Builder1 : S-Function  InitFcn=try, set_param(gcb,'FunctionName','LPMS_BE2_UART'), end  FunctionName=LPMS_BE2_UART  SFunctionModules=LPMS_BE2_UART_wrapper  SFunctionDeploymentMode=off  EnableBusSupport=off  mask(S-Function Builder){}
      mask help: Simulink:masks:SFunctionBuilder_MD
      mask init: same as hoppingControl/state estimation/S-Function Builder
      settings: CopyFcn=set_param(gcbh,'LinkStatus','none')  PreSaveFcn=try, set_param(gcb,'FunctionName','LPMS_BE2_UART'), end  OpenFcn=sfunctionwizard(gcbh)
      mask Display: plot(val(:,1),val(:,2)),disp(sys), port_label('output',1,'config'), port_label('output',2,'acc'), port_label('output',3,'gyr'), port_label('output',4,'mag'), port_label('output',5,'quat'), port_label('output',6,'euler'), port_label('output',7,'lin_acc'), port_label('output',8,'temp'), port_label('output',9,'time'), port_label('output',10,'ang')
  S-Function Builder2 : S-Function  Commented=on  InitFcn=try, set_param(gcb,'FunctionName','LPMS_BE2_SPI'), end  FunctionName=LPMS_BE2_SPI  SFunctionModules=LPMS_BE2_SPI_wrapper  SFunctionDeploymentMode=off  EnableBusSupport=off  mask(S-Function Builder){}
      mask help: Simulink:masks:SFunctionBuilder_MD
      mask init: same as hoppingControl/state estimation/S-Function Builder
      settings: CopyFcn=set_param(gcbh,'LinkStatus','none')  PreSaveFcn=try, set_param(gcb,'FunctionName','LPMS_BE2_SPI'), end  OpenFcn=sfunctionwizard(gcbh)
      mask Display: plot(val(:,1),val(:,2)),disp(sys), port_label('output',1,'config'), port_label('output',2,'acc'), port_label('output',3,'gyro'), port_label('output',4,'mag'), port_label('output',5,'quat'), port_label('output',6,'euler'), port_label('output',7,'lin_acc'), port_label('output',8,'temp'), port_label('output',9,'time')
  Saturation : Saturate  UpperLimit=2000  LowerLimit=-2000
  Saturation1 : Saturate  UpperLimit=16  LowerLimit=-16
  Saturation2 : Saturate  UpperLimit=10  LowerLimit=-10
  Saturation3 : Saturate  UpperLimit=1  LowerLimit=0
  Scope{,1..2,5,7..8,16,18..19,22,24..25,30} (13 alike) : Scope
  Scope{11..14} (4 alike) : Scope  Commented=on  NumInputPorts=2
  Scope15 : Scope  Commented=on
  Scope17 : Scope  Commented=on
  Scope27 : Scope  NumInputPorts=2
  Scope29 : Scope  NumInputPorts=2
  Scope6 : Scope  Commented=on
  Selector : Selector  InputPortWidth=7  IndexOptions=Index vector (dialog)  Indices=[1 2 3]  OutputSizes=1
  Selector1 : Selector  InputPortWidth=7  IndexOptions=Index vector (dialog)  Indices=[4 5 6]  OutputSizes=1
  Selector2 : Selector  InputPortWidth=7  IndexOptions=Index vector (dialog)  Indices=[7]  OutputSizes=1
  Selector4 : Selector  InputPortWidth=1  IndexOptions=Index vector (dialog)  Indices=[1]  OutputSizes=1
  Selector5 : Selector  InputPortWidth=3  IndexOptions=Index vector (dialog)  Indices=[2]  OutputSizes=1
  Selector6 : Selector  InputPortWidth=3  IndexOptions=Index vector (dialog)  Indices=[2]  OutputSizes=1
  Selector7 : Selector  InputPortWidth=4  IndexOptions=Index vector (dialog)  Indices=[2]  OutputSizes=1
  Signal Specification : SignalSpecification  Commented=through  Dimensions=3
  Signal Specification1 : SignalSpecification  Dimensions=4
  Sum2 : Sum  Inputs=+-
  Sum3 : Sum  Inputs=+-
  Switch : Switch  Criteria=u2 > Threshold
  UDP Receive : embdlinuxlib/UDP Receive  localURL='0.0.0.0'  localPort=31415  remoteURL='0.0.0.0'  remotePort=-1  recvBufferSize=8192  signalDatatype=single  dims=7  isVarSize=off  showBlockingTime=off  blockingTime=0  sampletime=-1  blockPlatform=Raspberry Pi
      settings: SourceProductName=Simulink Support Package for Raspberry Pi Hardware  SourceProductBaseCode=RASPPI
  Weighted Sample Time : SampleTimeMath  TsampMathOp=*
  Weighted Sample Time1 : SampleTimeMath  TsampMathOp=*
  Weighted Sample Time2 : SampleTimeMath  TsampMathOp=*
  Velocity : Outport
  Quaternion : Outport  Port=2
  Angular Velocity : Outport  Port=3
  Vicon Velocity : Outport  Port=4
  Vicon Quaternion : Outport  Port=5
  Pos : Outport  Port=6
  hAng : Outport  Port=7
  raw vicon data : Outport  Port=8
  estimated_data : Outport  Port=9
  wires:
  UDP Receive/1 -> Rate Transition/1
  Selector/1 -> [vicon_orient]
  Cast To Double3/1 -> Selector2/1, raw vicon data/1, Selector/1, Selector1/1
  Cast To Double2/1 -> Scope17/1, Add Constant1/1
  Selector2/1 -> Scope25/1, Gain7/1, Display1/1
  Weighted Sample Time/1 -> MATLAB Function/2(angVelInc)
  Rate Transition/1 -> Cast To Double3/1
  Weighted Sample Time1/1 -> MATLAB Function/1(velInc)
  S-Function Builder1/2 -> Saturation1/1
  S-Function Builder2/9 -> Display6/1
  Selector1/1 -> [vicon_pos]
  MATLAB Function/2(orient) -> Scope6/1, Scope27/2, Demux3/1, Manual Switch/2
  MATLAB Function/3(realAngVel) -> Manual Switch2/2, Scope7/1
  MATLAB Function/4(vVel) -> Signal Specification/1
  MATLAB Function/5(vOrient) -> Signal Specification1/1
  [reset] -> MATLAB Function/9(orientReset)
  Mux2/1 -> Manual Switch1/2, Scope5/1
  velLambda/1 -> MATLAB Function/6(velLambda)
  orientLambda/1 -> MATLAB Function/7(orientLambda)
  Arm length/1 -> MATLAB Function1/6(arm_length)
  Manual Switch12/1 -> Selector6/1, Display7/1, [pos_2D]
  MATLAB Function1/4(new_orient) -> Scope2/1, [quat_2D]
  MATLAB Function1/5(new_realAngVel) -> Demux/1
  Moving Average2/1 -> Mux/2
  Demux/2 -> Gain10/1
  Demux/1 -> Gain6/1
  Mux/1 -> Scope1/1, [ang_vel_2D]
  Moving Average3/1 -> Mux/1
  Demux1/3 -> Mux1/3
  Demux1/2 -> Moving Average5/1
  Demux1/1 -> Moving Average6/1
  Moving Average5/1 -> Mux1/2
  Moving Average6/1 -> Mux1/1
  Constant3/1 -> Moving Average3/2, Moving Average2/2, Moving Average1/2
  Demux/3 -> Gain11/1
  Moving Average1/1 -> Mux/3
  Demux3/4 -> Gain5/1
  Demux2/4 -> Scope11/1
  Demux2/3 -> Scope12/1
  Demux3/1 -> Scope14/2
  Demux2/2 -> Scope13/1
  Demux2/1 -> Scope14/1
  Demux3/2 -> Scope13/2
  Gain4/1 -> Scope12/2
  Demux3/3 -> Gain4/1
  Gain5/1 -> Scope11/2
  flipping/1 -> Switch/2
  Switch/1 -> Memory/1, [vicon_time]
  Memory/1 -> Switch/1
  S-Function Builder1/3 -> Saturation/1
  Saturation/1 -> Cast To Double2/1
  Saturation1/1 -> Cast To Double4/1
  Manual Switch1/1 -> ?
  Constant19/1 -> Manual Switch/1
  Manual Switch/1 -> ?
  Constant18/1 -> Manual Switch2/1
  Manual Switch2/1 -> ?
  Mux3/1 -> Manual Switch1/1
  MATLAB Function/6(vPos) -> ?
  MATLAB Function/1(vel) -> Demux4/1
  Moving Average4/1 -> Mux2/2
  Moving Average/1 -> Mux2/1
  Demux4/3 -> Mux2/3, Mux3/3
  Demux4/1 -> Low-Pass Filter (Discrete or Continuous)/1, Moving Average/1
  Constant17/1 -> Moving Average4/2, Moving Average/2
  Demux4/2 -> Low-Pass Filter (Discrete or Continuous)1/1, Moving Average4/1
  Low-Pass Filter (Discrete or Continuous)/1 -> Mux3/1
  Low-Pass Filter (Discrete or Continuous)1/1 -> Mux3/2
  Manual Switch3/1 -> MATLAB Function2/1(imu_accel)
  Saturation3/1 -> MATLAB Function2/5(accel_weight)
  Mux4/1 -> Scope/1
  Saturation2/1 -> Mux4/3
  Constant21/1 -> Gain13/1
  MATLAB Function2/7(debug) -> Scope8/1
  MATLAB Function2/1(estimate_pAng) -> Selector4/1, Display/1, Radians to Degrees3/1
  Radians to Degrees1/1 -> Manual Switch5/2
  Manual Switch5/1 -> MATLAB Function1/7(pAng)
  Selector4/1 -> Radians to Degrees1/1
  Gain13/1 -> MATLAB Function2/8(bound)
  Manual Switch6/1 -> Manual Switch3/1
  Low-Pass Filter (Discrete or Continuous)2/1 -> Manual Switch6/1
  Mux5/1 -> Manual Switch6/2
  Moving Average9/1 -> Mux5/3
  Moving Average8/1 -> Mux5/2
  Moving Average7/1 -> Mux5/1
  Demux5/2 -> Moving Average8/1
  Demux5/1 -> Moving Average7/1
  Demux5/3 -> Moving Average9/1
  Constant25/1 -> Moving Average9/2, Moving Average8/2, Moving Average7/2
  Radians to Degrees3/1 -> Mux4/2, [pAng_estimate]
  foot_pos/1 -> [foot_pos]
  Manual Switch11/1 -> Display8/1, [vel_2D], Scope19/1
  Signal Specification/1 -> Vicon Velocity/1
  Signal Specification1/1 -> Vicon Quaternion/1
  reset/1 -> [reset]
  [reset] -> MATLAB Function1/5(orient_reset)
  [reset] -> MATLAB Function2/6(orient_reset)
  Constant12/1 -> Moving Average6/2, Moving Average5/2
  foot_vel/1 -> [foot_vel]
  Constant13/1 -> MATLAB Function1/9(vel_weight)
  Manual Switch4/1 -> Velocity/1
  Manual Switch7/1 -> Pos/1
  Mux10/1 -> Scope24/1
  Selector5/1 -> Mux10/2
  Selector6/1 -> Sum2/1
  Sum2/1 -> Mux10/1
  Constant14/1 -> Sum2/2
  Selector7/1 -> hAng/1
  MATLAB Function1/8(debug) -> Selector7/1, Display4/1
  Constant20/1 -> Saturation3/1
  Manual Switch8/1 -> Quaternion/1
  state/1 -> [state]
  [foot_pos] -> MATLAB Function1/3(foot_pos)
  [foot_pos] -> MATLAB Function2/3(foot_pos)
  [foot_vel] -> MATLAB Function1/4(foot_vel)
  [foot_vel] -> MATLAB Function2/4(foot_vel)
  [state] -> MATLAB Function1/8(state)
  [state] -> MATLAB Function2/7(state)
  [state] -> Saturation2/1
  [pos_estimate] -> Selector5/1
  [pos_estimate] -> Manual Switch7/2
  MATLAB Function2/2(quat_orient) -> [quat_estimate]
  [quat_estimate] -> Scope27/1, Demux2/1
  [quat_estimate] -> Manual Switch8/2
  Manual Switch9/1 -> Angular Velocity/1
  [imu_ang_vel] -> Manual Switch9/2
  MATLAB Function2/4(estimate_vel) -> [vel_estimate], Scope22/1
  [vel_estimate] -> Manual Switch4/2
  Constant2/1 -> MATLAB Function2/9(arm_length)
  MATLAB Function2/3(ang_vel) -> [imu_ang_vel]
  Add Constant1/1 -> Gain8/1
  Add Constant/1 -> Gain12/1
  Cast To Double4/1 -> Scope15/1, Add Constant/1
  [vicon_pos] -> MATLAB Function/4(viconPos)
  [vicon_orient] -> MATLAB Function/5(viconOrient)
  Gain7/1 -> Switch/3
  [vicon_time] -> MATLAB Function/8(viconTime)
  Constant16/1 -> MATLAB Function2/10(vicon_flag)
  [vicon_pos] -> MATLAB Function2/13(vicon_pos)
  [vicon_orient] -> MATLAB Function2/14(vicon_orient)
  [vicon_time] -> MATLAB Function2/15(vicon_time)
  Constant23/1 -> MATLAB Function2/11(orient_lambda)
  Constant24/1 -> MATLAB Function2/12(vel_lambda)
  MATLAB Function2/5(estimate_pos) -> Scope29/1, Manual Switch10/1
  MATLAB Function2/6(mapped_vicon_pos) -> Manual Switch10/2, Scope29/2
  Manual Switch10/1 -> [pos_estimate], Display9/1
  S-Function Builder1/10 -> Cast To Double1/1, Display10/1, Scope30/1
  [imu_accel] -> Weighted Sample Time1/1
  Gain12/1 -> Scope16/1, [imu_accel]
  [imu_accel] -> Manual Switch3/2, Demux5/1, Low-Pass Filter (Discrete or Continuous)2/1
  Gain8/1 -> Scope18/1, [imu_gyro]
  [imu_gyro] -> MATLAB Function/3(angVel), Weighted Sample Time/1
  [imu_gyro] -> MATLAB Function1/2(imu_gyro)
  [imu_accel] -> Weighted Sample Time2/1
  Weighted Sample Time2/1 -> MATLAB Function1/1(velInc)
  [imu_gyro] -> MATLAB Function2/2(imu_gyro)
  Gain6/1 -> Moving Average3/1
  Gain10/1 -> Moving Average2/1
  Gain11/1 -> Moving Average1/1
  Cast To Double1/1 -> [encoder_ang]
  Gain14/1 -> Sum3/1
  Constant15/1 -> Sum3/2
  [encoder_ang] -> Gain14/1
  Mux6/1 -> estimated_data/1
  [quat_2D] -> Manual Switch8/1
  [ang_vel_2D] -> Manual Switch9/1
  [pos_2D] -> Manual Switch7/1
  [vel_2D] -> Manual Switch4/1
  Sum3/1 -> Display5/1, Manual Switch5/1, Mux4/1, [pAng_encoder]
  [vel_2D] -> Mux6/1
  [vel_estimate] -> Mux6/2
  [quat_2D] -> Mux6/3
  [quat_estimate] -> Mux6/4
  [ang_vel_2D] -> Mux6/5
  [imu_ang_vel] -> Mux6/6
  [pos_2D] -> Mux6/7
  [pos_estimate] -> Mux6/8
  [pAng_encoder] -> Mux6/9
  [pAng_estimate] -> Mux6/10
  MATLAB Function1/3(estimate_vel) -> Manual Switch11/2
  Mux1/1 -> Manual Switch11/1
  MATLAB Function1/1(new_vel) -> Demux1/1
  MATLAB Function1/6(new_vPos) -> Manual Switch12/1
  MATLAB Function1/7(ePos) -> Manual Switch12/2

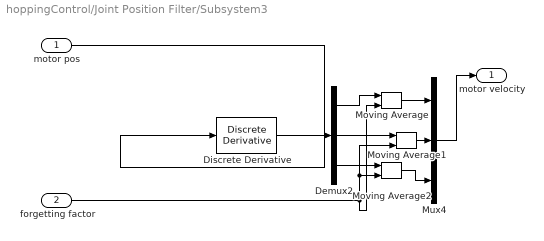
== system hoppingControl/Joint Position Filter/Subsystem3 ==
  motor pos : Inport
  forgetting factor : Inport  Port=2
  Demux2 : Demux  Outputs=3
  Discrete Derivative : simulink/Discrete/Discrete Derivative  gainval=1.0  ICPrevScaledInput=0.0  OutMin=[]  OutMax=[]  OutDataType=fixdt(1, 16)  OutScaling=2^-10  DoSatur=off
  Moving Average : dspstat3/Moving Average  Method=Exponential weighting  ForgettingFactorPort=on  SpecifyWindowLength=on  WindowLength=4  ForgettingFactor=0.2  SimulateUsing=Code generation
  Moving Average1 : dspstat3/Moving Average  Method=Exponential weighting  ForgettingFactorPort=on  SpecifyWindowLength=on  WindowLength=5  ForgettingFactor=0.2  SimulateUsing=Code generation
  Moving Average2 : dspstat3/Moving Average  Method=Exponential weighting  ForgettingFactorPort=on  SpecifyWindowLength=on  WindowLength=5  ForgettingFactor=0.2  SimulateUsing=Code generation
  Mux4 : Mux  Inputs=3
  "motor velocity " : Outport
  wires:
  Moving Average/1 -> Mux4/1
  Demux2/1 -> Moving Average/1
  Moving Average2/1 -> Mux4/3
  Mux4/1 -> "motor velocity "/1
  Demux2/3 -> Moving Average2/1
  Demux2/2 -> Moving Average1/1
  forgetting factor/1 -> Moving Average/2, Moving Average2/2, Moving Average1/2
  Moving Average1/1 -> Mux4/2
  Discrete Derivative/1 -> Demux2/1
  motor pos/1 -> Discrete Derivative/1

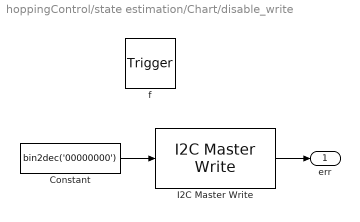
== system hoppingControl/state estimation/Chart/disable_write ==
  f : TriggerPort  TriggerType=function-call  VariantControl=(inherit)
      settings: CopyFcn=Stateflow.SLINSF.SimulinkMan.removeBlockPreDeleteFcn  PreDeleteFcn=Stateflow.SLINSF.SimulinkMan.unsafePredeleteFcn
  Constant : Constant  Value=bin2dec('00000000')
  I2C Master Write : raspberrypilib/I2C Master Write  BoardProperty=Pi 2 Model B  Mode=Master  SlaveAddress=hex2dec('32')  SlaveByteOrder=BigEndian  Direction=Transmitter  RegisterAddressMode=on  RegisterAddress=1  SlaveDataType=uint8  DataLength=1  NoAck=off  RepeatedStart=off  OutputStatus=on
      settings: SourceProductName=Simulink Support Package for Raspberry Pi Hardware  SourceProductBaseCode=RASPPI
  err : Outport
  wires:
  Constant/1 -> I2C Master Write/1
  I2C Master Write/1 -> err/1

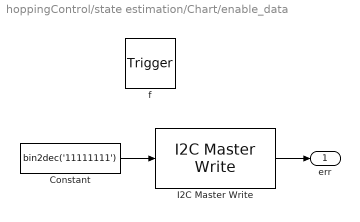
== system hoppingControl/state estimation/Chart/enable_data ==
  f : TriggerPort  TriggerType=function-call  VariantControl=(inherit)
      settings: CopyFcn=Stateflow.SLINSF.SimulinkMan.removeBlockPreDeleteFcn  PreDeleteFcn=Stateflow.SLINSF.SimulinkMan.unsafePredeleteFcn
  Constant : Constant  Value=bin2dec('11111111')
  I2C Master Write : raspberrypilib/I2C Master Write  BoardProperty=Pi 2 Model B  Mode=Master  SlaveAddress=hex2dec('32')  SlaveByteOrder=BigEndian  Direction=Transmitter  RegisterAddressMode=on  RegisterAddress=4  SlaveDataType=uint8  DataLength=1  NoAck=off  RepeatedStart=off  OutputStatus=on
      settings: SourceProductName=Simulink Support Package for Raspberry Pi Hardware  SourceProductBaseCode=RASPPI
  err : Outport
  wires:
  Constant/1 -> I2C Master Write/1
  I2C Master Write/1 -> err/1

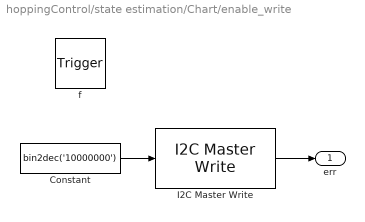
== system hoppingControl/state estimation/Chart/enable_write ==
  f : TriggerPort  TriggerType=function-call  VariantControl=(inherit)
      settings: CopyFcn=Stateflow.SLINSF.SimulinkMan.removeBlockPreDeleteFcn  PreDeleteFcn=Stateflow.SLINSF.SimulinkMan.unsafePredeleteFcn
  Constant : Constant  Value=bin2dec('10000000')
  I2C Master Write : raspberrypilib/I2C Master Write  BoardProperty=Pi 2 Model B  Mode=Master  SlaveAddress=hex2dec('32')  SlaveByteOrder=BigEndian  Direction=Transmitter  RegisterAddressMode=on  RegisterAddress=1  SlaveDataType=uint8  DataLength=1  NoAck=off  RepeatedStart=off  OutputStatus=on
      settings: SourceProductName=Simulink Support Package for Raspberry Pi Hardware  SourceProductBaseCode=RASPPI
  err : Outport
  wires:
  I2C Master Write/1 -> err/1
  Constant/1 -> I2C Master Write/1

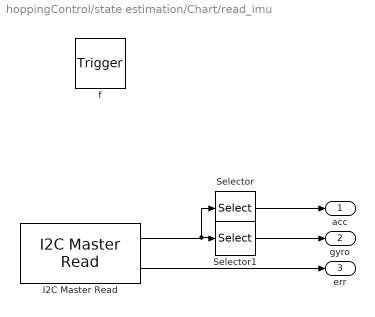
== system hoppingControl/state estimation/Chart/read_imu ==
  f : TriggerPort  TriggerType=function-call  VariantControl=(inherit)
      settings: CopyFcn=Stateflow.SLINSF.SimulinkMan.removeBlockPreDeleteFcn  PreDeleteFcn=Stateflow.SLINSF.SimulinkMan.unsafePredeleteFcn
  I2C Master Read : raspberrypilib/I2C Master Read  BoardProperty=Pi 2 Model B  Mode=Master  SlaveAddress=hex2dec('32')  SlaveByteOrder=LittleEndian  Direction=Receiver  RegisterAddressMode=on  RegisterAddress=hex2dec('24')  SlaveDataType=single  DataLength=6  NoAck=off  RepeatedStart=off  OutputStatus=on  SampleTime=-1
      settings: SourceProductName=Simulink Support Package for Raspberry Pi Hardware  SourceProductBaseCode=RASPPI
  Selector : Selector  InputPortWidth=6  IndexOptions=Index vector (dialog)  Indices=[1 2 3]  OutputSizes=1
  Selector1 : Selector  InputPortWidth=6  IndexOptions=Index vector (dialog)  Indices=[4 5 6]  OutputSizes=1
  acc : Outport
  gyro : Outport  Port=2
  err : Outport  Port=3
  wires:
  I2C Master Read/1 -> Selector1/1, Selector/1
  Selector/1 -> acc/1
  Selector1/1 -> gyro/1
  I2C Master Read/2 -> err/1

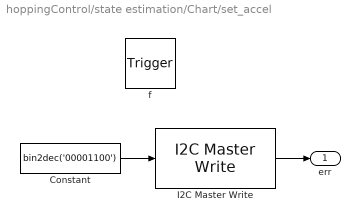
== system hoppingControl/state estimation/Chart/set_accel ==
  f : TriggerPort  TriggerType=function-call  VariantControl=(inherit)
      settings: CopyFcn=Stateflow.SLINSF.SimulinkMan.removeBlockPreDeleteFcn  PreDeleteFcn=Stateflow.SLINSF.SimulinkMan.unsafePredeleteFcn
  Constant : Constant  Value=bin2dec('00001100')
  I2C Master Write : raspberrypilib/I2C Master Write  BoardProperty=Pi 2 Model B  Mode=Master  SlaveAddress=hex2dec('32')  SlaveByteOrder=BigEndian  Direction=Transmitter  RegisterAddressMode=on  RegisterAddress=5  SlaveDataType=uint8  DataLength=1  NoAck=off  RepeatedStart=off  OutputStatus=on
      settings: SourceProductName=Simulink Support Package for Raspberry Pi Hardware  SourceProductBaseCode=RASPPI
  err : Outport
  wires:
  Constant/1 -> I2C Master Write/1
  I2C Master Write/1 -> err/1

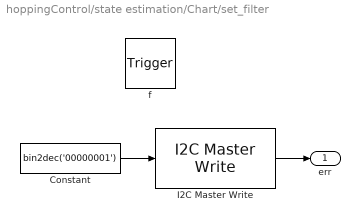
== system hoppingControl/state estimation/Chart/set_filter ==
  f : TriggerPort  TriggerType=function-call  VariantControl=(inherit)
      settings: CopyFcn=Stateflow.SLINSF.SimulinkMan.removeBlockPreDeleteFcn  PreDeleteFcn=Stateflow.SLINSF.SimulinkMan.unsafePredeleteFcn
  Constant : Constant  Value=bin2dec('00000001')
  I2C Master Write : raspberrypilib/I2C Master Write  BoardProperty=Pi 2 Model B  Mode=Master  SlaveAddress=hex2dec('32')  SlaveByteOrder=BigEndian  Direction=Transmitter  RegisterAddressMode=on  RegisterAddress=7  SlaveDataType=uint8  DataLength=1  NoAck=off  RepeatedStart=off  OutputStatus=on
      settings: SourceProductName=Simulink Support Package for Raspberry Pi Hardware  SourceProductBaseCode=RASPPI
  err : Outport
  wires:
  Constant/1 -> I2C Master Write/1
  I2C Master Write/1 -> err/1

== system hoppingControl/state estimation/Chart/set_freq ==
  f : TriggerPort  TriggerType=function-call  VariantControl=(inherit)
      settings: CopyFcn=Stateflow.SLINSF.SimulinkMan.removeBlockPreDeleteFcn  PreDeleteFcn=Stateflow.SLINSF.SimulinkMan.unsafePredeleteFcn
  Constant : Constant  Value=bin2dec('00000101')
  I2C Master Write : raspberrypilib/I2C Master Write  BoardProperty=Pi 2 Model B  Mode=Master  SlaveAddress=hex2dec('32')  SlaveByteOrder=BigEndian  Direction=Transmitter  RegisterAddressMode=on  RegisterAddress=3  SlaveDataType=uint8  DataLength=1  NoAck=off  RepeatedStart=off  OutputStatus=on
      settings: SourceProductName=Simulink Support Package for Raspberry Pi Hardware  SourceProductBaseCode=RASPPI
  err : Outport
  wires:
  Constant/1 -> I2C Master Write/1
  I2C Master Write/1 -> err/1

== system hoppingControl/state estimation/Chart/set_gyro ==
  f : TriggerPort  TriggerType=function-call  VariantControl=(inherit)
      settings: CopyFcn=Stateflow.SLINSF.SimulinkMan.removeBlockPreDeleteFcn  PreDeleteFcn=Stateflow.SLINSF.SimulinkMan.unsafePredeleteFcn
  Constant : Constant  Value=bin2dec('00001000')
  I2C Master Write : raspberrypilib/I2C Master Write  BoardProperty=Pi 2 Model B  Mode=Master  SlaveAddress=hex2dec('32')  SlaveByteOrder=BigEndian  Direction=Transmitter  RegisterAddressMode=on  RegisterAddress=6  SlaveDataType=uint8  DataLength=1  NoAck=off  RepeatedStart=off  OutputStatus=on
      settings: SourceProductName=Simulink Support Package for Raspberry Pi Hardware  SourceProductBaseCode=RASPPI
  err : Outport
  wires:
  Constant/1 -> I2C Master Write/1
  I2C Master Write/1 -> err/1
